simulink library "Sim_Library"  (R2015b)
settings: Solver=ode45  SolverMode=SingleTasking  StartTime=0.0  StopTime=10.0  RelTol=1e-3
undefined symbols (not defined in the file): agent, CTRL, FRAME, k, k_throttle, l, ROTOR
libraries: Sim_Library x17, vrlib x2, aerolibutil x1
(part 1 of 2)
settings Model: Creator=sgjdouth  LastModifiedBy=uos
settings DataIOCC: SaveFormat=Array
settings OptimizationCC: BlockReduction=off  BooleanDataType=off
settings DebuggingCC: SaveWithParameterizedLinksMsg=none  UnderspecifiedInitializationDetection=Classic  MergeDetectMultiDrivingBlocksExec=none  SignalResolutionControl=TryResolveAllWithWarning  StrictBusMsg=Warning
settings HardwareCC: ProdBitPerPointer=32  ProdLargestAtomicFloat=None  ProdIntDivRoundTo=Undefined  ProdEndianess=Unspecified  ProdWordSize=32  ProdHWDeviceType=32-bit Generic  TargetUnknown=on
settings GRTTargetCC: GeneratePreprocessorConditionals=Disable all
settings ConfigComp: CovModelRefEnable=Off  CovSFcnEnable=off

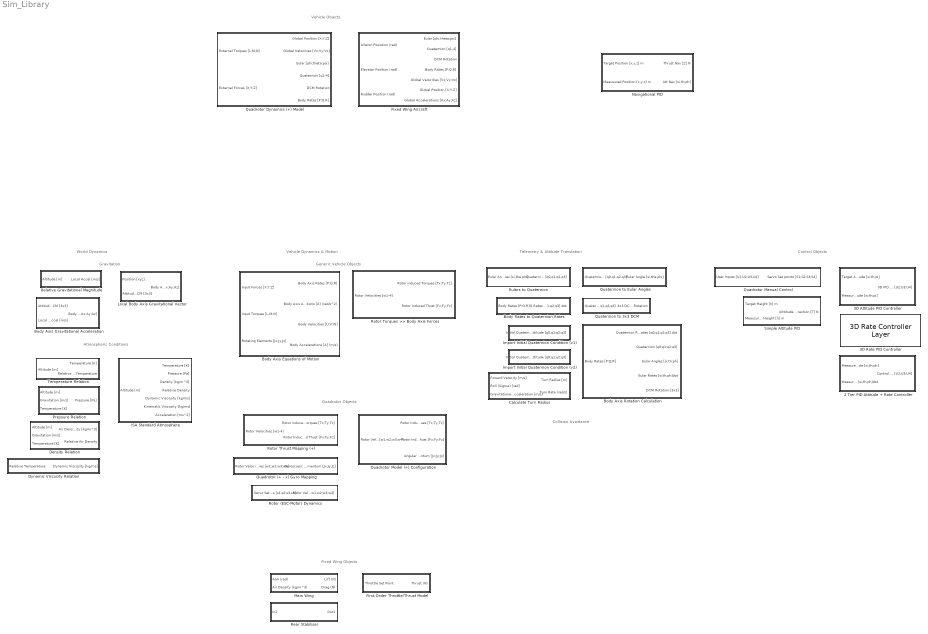
== system Sim_Library ==
  note: Gravitation
  note: Telemetry & Attitude Translation
  note: Vehicle Dynamics & Motion
  note: Control Objects
  note: World Dynamics
  note: Atmospheric Conditions
  note: Generic Vehicle Objects
  note: Quadrotor Objects
  note: Fixed Wing Objects
  note: Vehicle Objects
  note: Collision Avoidance
  2 Tier PID Attitude + Rate Controller : Subsystem
      mask Display:
      | port_label ('input',1,'IMU Attitude [\phi;\theta;\psi]','TexMode','on')
      | port_label ('input',2,'IMU Rates [\phi;\theta;\psi]dot','TexMode','on')
      | port_label ('output',1,'Control Correction [U_{2-4}]','TexMode','on')
  3D Attitude PID Controller : Subsystem
      mask Display:
      | port_label ('input',1,'Target Attitude [\phi;\theta;\psi]','TexMode','on')
      | port_label ('input',2,'Measured Attitude [\phi;\theta;\psi]','TexMode','on')
      | port_label ('output',1,'Attitude Correction [U_{2-4}]','TexMode','on')
  3D Rate PID Controller : Sim_Library/2 Tier PID Attitude + Rate Controller/3D Rate Controller Layer  SystemSampleTime=-1
  Body Axis Equations of Motion : Subsystem
      mask Display:
      | image('Sim_masks/3D_block_model.jpg')
      | port_label ('input', 1,'Net Forces [F_{x};F_{y};F_{z}]','TexMode','on')
      | port_label ('input', 2,'Net Torques [{\tau}_{L};{\tau}_{M};{\tau}_{N}]','TexMode','on')
      | port_label ('input', 3,'Rotating Elements [J_{x};J_{y};J_{z}]','TexMode','on')
      | port_label ('output',1,'Axis Rates [P;Q:R]','TexMode','on')
      | port_label ('output',2,'Angular Acceleration [omegaA]','TexMode','on')
      | port_label ('output',3,'Body Velocities [V_{x};V_{y};V_{z}]','TexMode','on')
      | port_label ('output',4,'Body Accelerations [A]','TexMode','on')
  Body Axis Gravitational Acceleration : Subsystem
      mask Display:
      | port_label ('input', 1,'Attitude DCM [3x3]','TexMode','on')
      | port_label ('input', 2,'Local Gravity [m/s]','TexMode','on')
      | port_label ('output',1,'Gravitation [g_{x};g_{y};g_{z}]','TexMode','on')
  "Body Axis Rotation Calculation " : Subsystem
      mask Display:
      | image('Sim_masks/Telemetry2.jpg')
      | port_label ('input', 1,'Body Rates [P;Q;R]','TexMode','on')
      | port_label ('output',1,'Quaternion Rates [q_{1-4}]','TexMode','on')
      | port_label ('output',2,'Quaternion [q_{1-4}]','TexMode','on')
      | port_label ('output',3,'Euler Angles [\phi;\theta;\psi]','TexMode','on')
      | port_label ('output',4,'Eular Rates [\phi;\theta;\psi]dot','TexMode','on')
      | port_label ('output',5,'DCM Rotation [3x3]')
  Body Rates to Quaternion Rates : Subsystem
      mask Display:
      | port_label ('input', 1,'Body Rates [p;q;r]','TexMode','on')
      | port_label ('output',1,'Q Rates [q_{1-4}]^{T}','TexMode','on')
  Calculate Turn Radius : Subsystem
      mask Display:
      | port_label ('input', 1,'Velocity (m/s)','TexMode','on')
      | port_label ('input', 2,'Roll Angle (rad)','TexMode','on')
      | port_label ('input', 3,'Local Gravitation (m/s)','TexMode','on')
      | port_label ('output',1,'Turn Radius (m)','TexMode','on')
      | port_label ('output',2,'Turn Rate (rad/s)','TexMode','on')
  Density Relation : Subsystem
  Dynamic Viscosity Relation : Subsystem
  Eulars to Quaternion : Subsystem
      mask Display:
      | port_label ('input', 1,'Eular Angles [\sigma;\theta;\phi]','TexMode','on')
      | port_label ('output',1,'Quaternion [q_{1-4}]^{T}','TexMode','on')
  First Order Throttle/Thrust Model : Subsystem
  Fixed Wing Aircraft : Subsystem
      mask Display:
      | image('Sim_masks/F16 wireframe.jpg');
      | port_label ('output',1,'Euler Angles [\phi;\theta;\psi]','TexMode','on');
      | port_label ('output',2,'Quaternion [q_{1-4}]','TexMode','on');
      | port_label ('output',3,'DCM Rotation [3x3]','TexMode','on');
      | port_label ('output',4,'Body Axis Rates [P;Q;R]','TexMode','on');
      | port_label ('output',5,'Velocities [V_{x},V_{y},V_{z}]','TexMode','on');
      | port_label ('output',6,'Position [x;y;z]','TexMode','on');
      | port_label ('input',1,'Velocity [V_{x};V_{y};V_{z}]','TexMode','on');
      | port_label ('input',2,'AoA (rad)','TexMode','on');
  ISA Standard Atmosphere : Subsystem
      mask Display:
      | port_label('input',1,'Altitude (m)','texmode','on')
      | port_label('output',1,'Temperature (K)','texmode','on')
      | port_label('output',2,'Pressure (Pa)','texmode','on')
      | port_label('output',3,'Density (kg/m^3)','texmode','on')
      | port_label('output',4,'Relative Density','texmode','on')
      | port_label('output',5,'Dynamic Viscosity (kg/ms)','texmode','on')
      | port_label('output',6,'Kinematic Viscosity (kg/ms)','texmode','on')
      | port_label('output',7,'Acceleration (ms^2)','texmode','on')
  Import Initial Quaternion Condition (v1) : Subsystem
      mask Display: port_label ('output',1,'Initial Quaternion [q_{1-4}]^{T}','TexMode','on')
  Import Initial Quaternion Condition (v2) : Subsystem
      mask Display: port_label ('output',1,'Initial Quaternion [q_{1-4}]^{T}','TexMode','on')
  Local Body Axis Gravitational Vector : Subsystem
      mask Display:
      | port_label ('input', 1,'Position [X;Y;Z]','TexMode','on')
      | port_label ('input', 2,'Attitude DCM [3x3]','TexMode','on')
      | port_label ('output',1,'Body Gravitation [g_{x};g_{y};g_{z}]','TexMode','on')
  "Main Wing " : Subsystem
  Navigational PID : Subsystem
  Pressure Relation : Subsystem
  Quadrotor (+ - x) Gyro Mapping : Subsystem
      mask Display:
      | port_label ('input', 1,'Rotor Velocities [{\omega}_{1-4}]^{T}','TexMode','on')
      | port_label ('output',1,'Rotor Momentum [J_{x};J_{y};J_{z}]','TexMode','on')
  Quadrotor Dynamics (+) Model : Subsystem
      mask Display:
      | image('Sim_masks/QuadMask+.jpg');
      | port_label ('output',1,'Euler Angles [\phi;\theta;\psi]','TexMode','on');
      | port_label ('output',2,'Quaternion [q_{1-4}]','TexMode','on');
      | port_label ('output',3,'DCM Rotation [3x3]','TexMode','on');
      | port_label ('output',4,'Body Axis Rates [P;Q;R]','TexMode','on');
      | port_label ('output',5,'Velocities [V_{x},V_{y},V_{z}]','TexMode','on');
      | port_label ('output',6,'Position [x;y;z]','TexMode','on');
      | port_label ('input',1,'Rotor Velocities [\omega_{1-4}]','TexMode','on');
      | port_label ('input',2,'External Torques [L;M;N]','TexMode','on');
      | port_label ('input',3,'External Forces [F_{x};F_{y};F_{z}]','TexMode','on');
  "Quadrotor Manual Control " : Subsystem
      mask Display:
      | port_label ('input',1,'Control Inputs [U_{1-4}]','TexMode','on')
      | port_label ('output',1,'Servo Set Points_{0-255} [S_{1-4}]','TexMode','on')
  Quadrotor Model (+) Configuration : Subsystem
      mask Display:
      | port_label ('input', 1,'Rotor Velocities [\omega_{1-4}]','TexMode','on')
      | port_label ('output',1,'Net Torques [\tau_{x},\tau_{y},\tau_{z}]','TexMode','on')
      | port_label ('output',2,'Net Thrust [F_{x},F_{y},F_{z}]','TexMode','on')
      | port_label ('output',3,'Angular Momentum [J_{x},J_{y},J_{z}]','TexMode','on')
  "Quaternion to 3x3 DCM " : Subsystem
      mask Display:
      | port_label ('input', 1,'Quaternion [q_{1-4}]^{T}','TexMode','on')
      | port_label ('output',1,'DCM [3x3]','TexMode','on')
  Quaternion to Eular Angles : Subsystem
      mask Display:
      | port_label ('input',1,'Quaternion [q_{1-4}]^{T}','TexMode','on')
      | port_label ('output',1,'Eular Angles [\sigma;\theta;\phi]','TexMode','on')
  Rear Stabiliser : Subsystem
  Relative Gravitational Magnitude : Subsystem
  Rotor (ESC-Motor) Dynamics : Subsystem
      mask Display:
      | port_label ('input', 1,'Servo CMD [S_{1-4}]','TexMode','on')
      | port_label ('output',1,'Rotational Rates [\omega_{1-4}]','TexMode','on')
  Rotor Thrust Mapping (+) : Subsystem
      mask Display:
      | port_label ('input', 1,'Rotor Velocities [\omega_{1-4}]','TexMode','on')
      | port_label ('output',1,'Rotor Induced Torques [\tau_{x},\tau_{y},\tau_{z}]','TexMode','on')
      | port_label ('output',2,'Rotor Induced Thrust [F_{x},F_{y},F_{z}]','TexMode','on')
  Rotor Torques >> Body Axis Forces : Subsystem
      mask Display:
      | image('Sim_masks/Body Arm Coordinates.jpg')
      | port_label ('input', 1,'Rotor Velocities [\omega_{1-N}]','TexMode','on')
      | port_label ('output',1,'Rotor Induced Torques [\tau_{x},\tau_{y},\tau_{z}]','TexMode','on')
      | port_label ('output',2,'Rotor Induced Thrust [F_{x},F_{y},F_{z}]','TexMode','on')
  Simple Altitude PID : Subsystem
      mask Display:
      | port_label ('input',1,'Target Altitude [m]','TexMode','on')
      | port_label ('input',2,'Measured Altitude [m]','TexMode','on')
      | port_label ('output',1,'Throttle Correction [U_{1}]','TexMode','on')
  Temperature Relation : Subsystem

== system Sim_Library/2 Tier PID Attitude + Rate Controller ==
  Measured Attitude [si;th;ph] : Inport
  Measured Rates [si;th;ph]dot : Inport  Port=2
  3D PID Controller (Attitude) : Sim_Library/3D PID Controller (Attitude)
  3D Rate Controller Layer : Subsystem
      mask Display:
      | port_label ('input',1,'Measured Rates [\phi;\theta;\psi]dot','TexMode','on')
      | port_label ('input',2,'Target Rates [\phi;\theta;\psi]dot','TexMode','on')
      | port_label ('output',1,'Attitude Correction [U_{2-4}]','TexMode','on')
  Hold Level Horizon : Constant  Value=[0;0;0]
  Control Outputs [U2;U3;U4] : Outport
  wires:
  3D Rate Controller Layer/1(PID Outputs [Ksi;Kth;Kpi]) -> Control Outputs [U2;U3;U4]/1
  Measured Rates [si;th;ph]dot/1 -> 3D Rate Controller Layer/1(Measured Rates [si;th;pi] dot)
  3D PID Controller (Attitude)/1 -> 3D Rate Controller Layer/2(Target Rates [si;th;pi] dot)
  Hold Level Horizon/1 -> 3D PID Controller (Attitude)/1
  Measured Attitude [si;th;ph]/1 -> 3D PID Controller (Attitude)/2

== system Sim_Library/3D Attitude PID Controller ==
  note: 3D PID Attitude Control Calculator
  Target Attitude [si;th;pi] : Inport
  Measured Attitude [si;th;pi] : Inport  Port=2
  Attitude Integrator : Integrator  InitialCondition=[0;0;0]
  Constant : Constant  Value=CTRL.kp  VectorParams1D=off
  Constant1 : Constant  Value=CTRL.kd  VectorParams1D=off
  Constant2 : Constant  Value=CTRL.ki  VectorParams1D=off
  D Gains [si,th,pi] : Product
  Derivative : Derivative
  Display : Display
  Display1 : Display
  I Gains [si,th,pi] : Product
  P Gains [si,th,pi] : Product
  Subtract : Sum  Inputs=-+
  Sum2 : Sum  Inputs=+++
  3D PID Outputs [U2;U3;U4] : Outport
  wires:
  Target Attitude [si;th;pi]/1 -> Subtract/2
  Measured Attitude [si;th;pi]/1 -> Display1/1, Subtract/1
  Sum2/1 -> 3D PID Outputs [U2;U3;U4]/1, Display/1
  Derivative/1 -> Sum2/3
  Subtract/1 -> D Gains [si,th,pi]/2, P Gains [si,th,pi]/2, I Gains [si,th,pi]/2
  Constant1/1 -> D Gains [si,th,pi]/1
  Constant/1 -> P Gains [si,th,pi]/1
  Constant2/1 -> I Gains [si,th,pi]/1
  D Gains [si,th,pi]/1 -> Derivative/1
  P Gains [si,th,pi]/1 -> Sum2/1
  Attitude Integrator/1 -> Sum2/2
  I Gains [si,th,pi]/1 -> Attitude Integrator/1

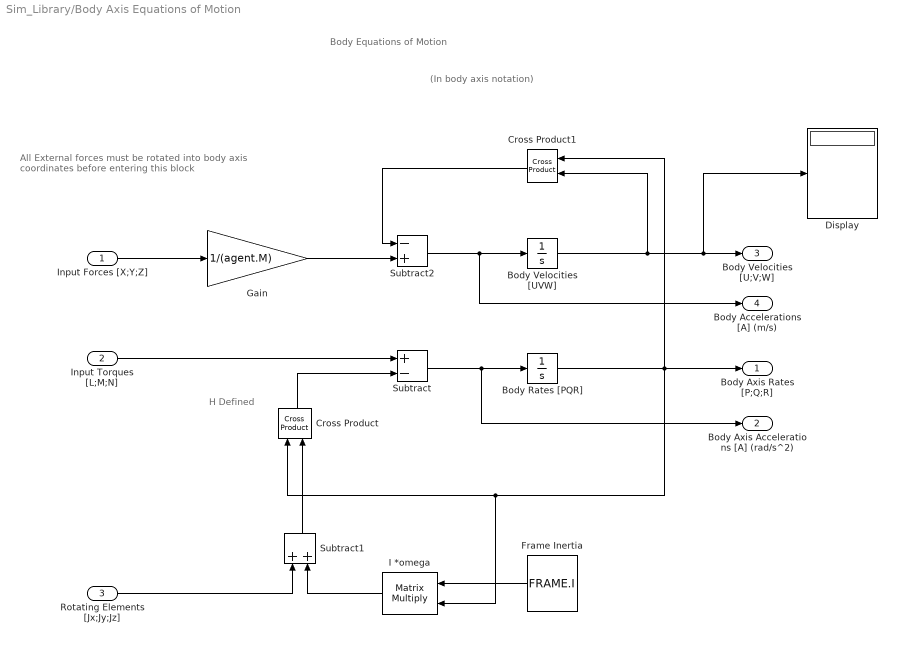
== system Sim_Library/Body Axis Equations of Motion ==
  note: All External forces must be rotated into
      | body axis coordinates before entering this block
  note: (In body axis notation)
  note: Body Equations of Motion
  note: H Defined
  Input Forces [X;Y;Z] : Inport
  Input Torques [L;M;N] : Inport  Port=2
  Rotating Elements [Jx;Jy;Jz] : Inport  Port=3
  Body Rates [PQR] : Integrator  InitialCondition=[0;0;0]
  Body Velocities [UVW] : Integrator  InitialCondition=[0;0;0]
  Cross Product : vrlib/Utilities/Cross Product
  Cross Product1 : vrlib/Utilities/Cross Product
  Display : Display
  Frame Inertia : Constant  Value=FRAME.I
  Gain : Gain  Gain=1/(agent.M)
  I *omega : Product  Multiplication=Matrix(*)
  Subtract : Sum  Inputs=+-
  Subtract1 : Sum
  Subtract2 : Sum  Inputs=-+
  Body Axis Rates [P;Q;R] : Outport
  Body Axis Accelerations [A] (rad/s^2) : Outport  Port=2
  Body Velocities [U;V;W] : Outport  Port=3
  Body Accelerations [A] (m/s) : Outport  Port=4
  wires:
  Gain/1 -> Subtract2/2
  Subtract2/1 -> Body Accelerations [A] (m/s)/1, Body Velocities [UVW]/1
  Cross Product1/1 -> Subtract2/1
  Body Velocities [UVW]/1 -> Display/1, Body Velocities [U;V;W]/1, Cross Product1/2
  Body Rates [PQR]/1 -> I *omega/2, Cross Product/1, Body Axis Rates [P;Q;R]/1, Cross Product1/1
  Frame Inertia/1 -> I *omega/1
  Subtract/1 -> Body Axis Accelerations [A] (rad/s^2)/1, Body Rates [PQR]/1
  Cross Product/1 -> Subtract/2
  I *omega/1 -> Subtract1/2
  Subtract1/1 -> Cross Product/2
  Input Forces [X;Y;Z]/1 -> Gain/1
  Input Torques [L;M;N]/1 -> Subtract/1
  Rotating Elements [Jx;Jy;Jz]/1 -> Subtract1/1

== system Sim_Library/Body Axis Gravitational Acceleration ==
  note: Gravitational Model
  note: Newtons equation of gravity, extended to provide a local gravitational vector
  note: Assumptions; Gravitational linearity, reference is Earth and down is positive.
  Attitude DCM [3x3] : Inport
  Local Gravitational Accel [m/s] : Inport  Port=2
  Gain : Gain  Gain=[0;0;1]
  Product1 : Product  Multiplication=Matrix(*)
  Body Accel [Ax;Ay;Az] : Outport
  wires:
  Gain/1 -> Product1/2
  Product1/1 -> Body Accel [Ax;Ay;Az]/1
  Attitude DCM [3x3]/1 -> Product1/1
  Local Gravitational Accel [m/s]/1 -> Gain/1

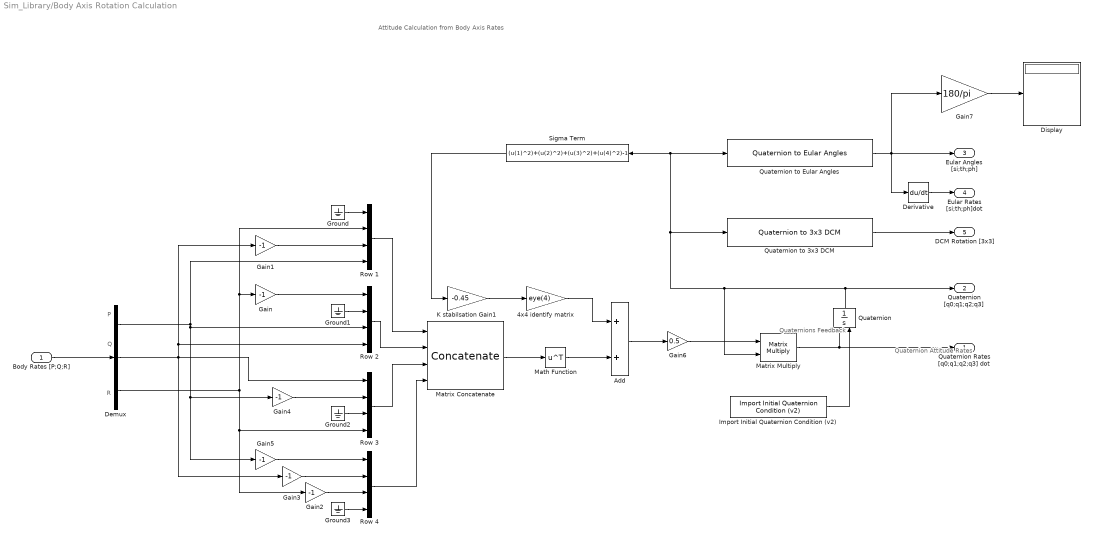
== system Sim_Library/Body Axis Rotation Calculation  ==
  note: R
  note: Q
  note: P
  note: Quaternions Feedback
  note: Attitude Calculation from Body Axis Rates
  note: Quaternion Attitude Rates
  Body Rates [P;Q;R] : Inport
  4x4 identify matrix : Gain  Gain=eye(4)
  Add : Sum
  Demux : Demux  Outputs=3
  Derivative : Derivative
  Display : Display
  Gain{,1..5} (6 alike) : Gain  Gain=-1
  Gain6 : Gain  Gain=0.5
  Gain7 : Gain  Gain=180/pi
  Ground{,1..3} (4 alike) : Ground
  Import Initial Quaternion Condition (v2) : Sim_Library/Import Initial Quaternion Condition (v2)  SystemSampleTime=-1
  K stabilsation Gain1 : Gain  Gain=-0.45
  Math Function : Math  Operator=transpose  SaturateOnIntegerOverflow=on
  Matrix Concatenate : Concatenate  NumInputs=4  Mode=Multidimensional array  ConcatenateDimension=2
  Matrix Multiply : Product  Multiplication=Matrix(*)
  Quaternion : Integrator  InitialConditionSource=external  InitialCondition=[0;0;0;1]  ZeroCross=off
  "Quaternion to 3x3 DCM " : Sim_Library/Quaternion to 3x3 DCM   SystemSampleTime=-1
  Quaternion to Eular Angles : Sim_Library/Quaternion to Eular Angles  SystemSampleTime=-1
  Row {1..4} (4 alike) : Concatenate  NumInputs=4
  Sigma Term : Fcn  Expr=(u(1)^2)+(u(2)^2)+(u(3)^2)+(u(4)^2)-1
  Quaternion Rates [q0;q1;q2;q3] dot : Outport
  Quaternion [q0;q1;q2;q3] : Outport  Port=2
  Eular Angles [si;th;ph] : Outport  Port=3
  Eular Rates [si;th;ph]dot : Outport  Port=4
  DCM Rotation [3x3] : Outport  Port=5
  wires:
  Math Function/1 -> Add/2
  Body Rates [P;Q;R]/1 -> Demux/1
  Gain7/1 -> Display/1
  K stabilsation Gain1/1 -> 4x4 identify matrix/1
  Add/1 -> Gain6/1
  4x4 identify matrix/1 -> Add/1
  Matrix Concatenate/1 -> Math Function/1
  Ground1/1 -> Row 2/2
  Ground2/1 -> Row 3/3
  Ground3/1 -> Row 4/4
  Ground/1 -> Row 1/1
  Gain5/1 -> Row 4/1
  Gain4/1 -> Row 3/2
  Demux/1 -> Row 2/3, Gain4/1, Gain5/1, Row 1/4
  Gain3/1 -> Row 4/2
  Gain1/1 -> Row 1/3
  Demux/2 -> Gain3/1, Row 3/1, Row 2/4, Gain1/1
  Gain2/1 -> Row 4/3
  Gain/1 -> Row 2/1
  Demux/3 -> Row 3/4, Gain2/1, Row 1/2, Gain/1
  Row 1/1 -> Matrix Concatenate/1
  Row 2/1 -> Matrix Concatenate/2
  Row 3/1 -> Matrix Concatenate/3
  Row 4/1 -> Matrix Concatenate/4
  Matrix Multiply/1 -> Quaternion Rates [q0;q1;q2;q3] dot/1, Quaternion/1
  Sigma Term/1 -> K stabilsation Gain1/1
  Gain6/1 -> Matrix Multiply/1
  Quaternion/1 -> Quaternion [q0;q1;q2;q3]/1, Quaternion to Eular Angles/1, Sigma Term/1, "Quaternion to 3x3 DCM "/1, Matrix Multiply/2
  "Quaternion to 3x3 DCM "/1 -> DCM Rotation [3x3]/1
  Quaternion to Eular Angles/1 -> Gain7/1, Derivative/1, Eular Angles [si;th;ph]/1
  Derivative/1 -> Eular Rates [si;th;ph]dot/1
  Import Initial Quaternion Condition (v2)/1 -> Quaternion/2

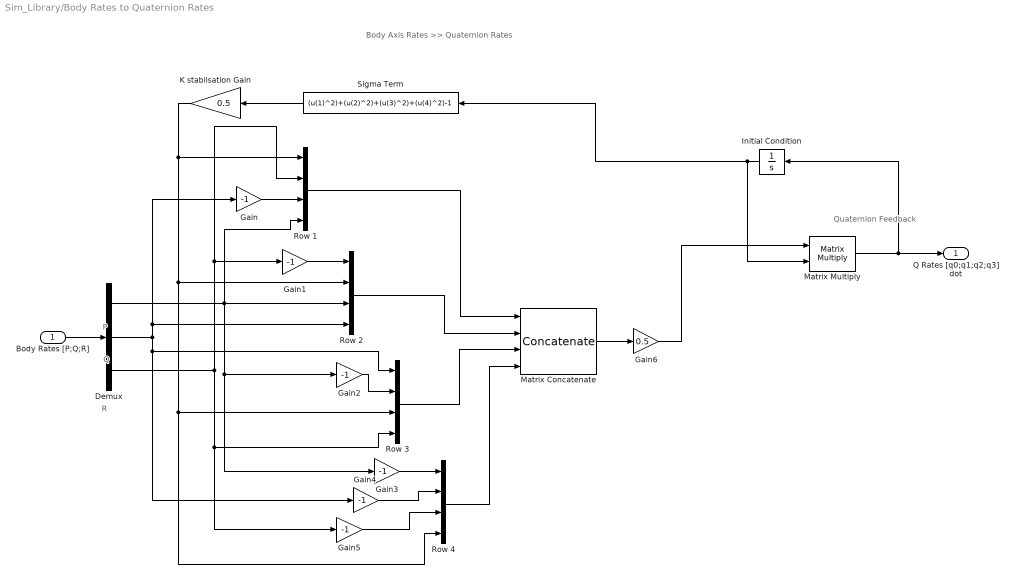
== system Sim_Library/Body Rates to Quaternion Rates ==
  note: Quaternion Feedback
  note: P
  note: Q
  note: R
  note: Body Axis Rates >> Quaternion Rates
  Body Rates [P;Q;R] : Inport
  Demux : Demux  Outputs=3
  Gain{,1..5} (6 alike) : Gain  Gain=-1
  Gain6 : Gain  Gain=0.5
  "Initial Condition " : Integrator  InitialCondition=[0;0;0]
  K stabilsation Gain : Gain  Gain=0.5
  Matrix Concatenate : Concatenate  NumInputs=4  Mode=Multidimensional array  ConcatenateDimension=2
  Matrix Multiply : Product  Multiplication=Matrix(*)
  Row {1..4} (4 alike) : Concatenate  NumInputs=4
  Sigma Term : Fcn  Expr=(u(1)^2)+(u(2)^2)+(u(3)^2)+(u(4)^2)-1
  Q Rates [q0;q1;q2;q3] dot : Outport
  wires:
  "Initial Condition "/1 -> Sigma Term/1, Matrix Multiply/2
  Gain6/1 -> Matrix Multiply/1
  K stabilsation Gain/1 -> Row 1/1, Row 2/2, Row 3/3, Row 4/4
  Sigma Term/1 -> K stabilsation Gain/1
  Matrix Multiply/1 -> Q Rates [q0;q1;q2;q3] dot/1, "Initial Condition "/1
  Matrix Concatenate/1 -> Gain6/1
  Row 4/1 -> Matrix Concatenate/4
  Row 3/1 -> Matrix Concatenate/3
  Row 2/1 -> Matrix Concatenate/2
  Row 1/1 -> Matrix Concatenate/1
  Gain5/1 -> Row 4/3
  Gain4/1 -> Row 4/2
  Gain3/1 -> Row 4/1
  Gain2/1 -> Row 3/2
  Gain1/1 -> Row 2/1
  Demux/1 -> Row 1/4, Row 2/3, Gain2/1, Gain3/1
  Demux/2 -> Gain/1, Row 2/4, Gain4/1, Row 3/1
  Gain/1 -> Row 1/3
  Demux/3 -> Gain1/1, Row 1/2, Row 3/4, Gain5/1
  Body Rates [P;Q;R]/1 -> Demux/1

== system Sim_Library/Calculate Turn Radius ==
  note: Turn Radius, R = V^2/(g*tan(sig))
  note: Calculate Turn Performance Parameters
  note: Yaw rate, Phi = (g*tan(sig))/V
  Foward Velocity [m/s] : Inport
  Roll (Sigma) [rad] : Inport  Port=2
  Gravitational Acceleration [m/s] : Inport  Port=3
  (g*tan(sig))/V : Product  Inputs=*/
  V^2 : Math  Operator=square  SaturateOnIntegerOverflow=on
  V^2/(g*tan(sig) : Product  Inputs=*/
  g*tan(sig) : Product
  tan(sig) : Trigonometry  Operator=tan
  Turn Radius [m] : Outport
  Turn Rate (rad/s) : Outport  Port=2
  wires:
  Foward Velocity [m/s]/1 -> (g*tan(sig))/V/2, V^2/1
  V^2/1 -> V^2/(g*tan(sig)/1
  Roll (Sigma) [rad]/1 -> tan(sig)/1
  tan(sig)/1 -> g*tan(sig)/1
  Gravitational Acceleration [m/s]/1 -> g*tan(sig)/2
  g*tan(sig)/1 -> V^2/(g*tan(sig)/2, (g*tan(sig))/V/1
  V^2/(g*tan(sig)/1 -> Turn Radius [m]/1
  (g*tan(sig))/V/1 -> Turn Rate (rad/s)/1

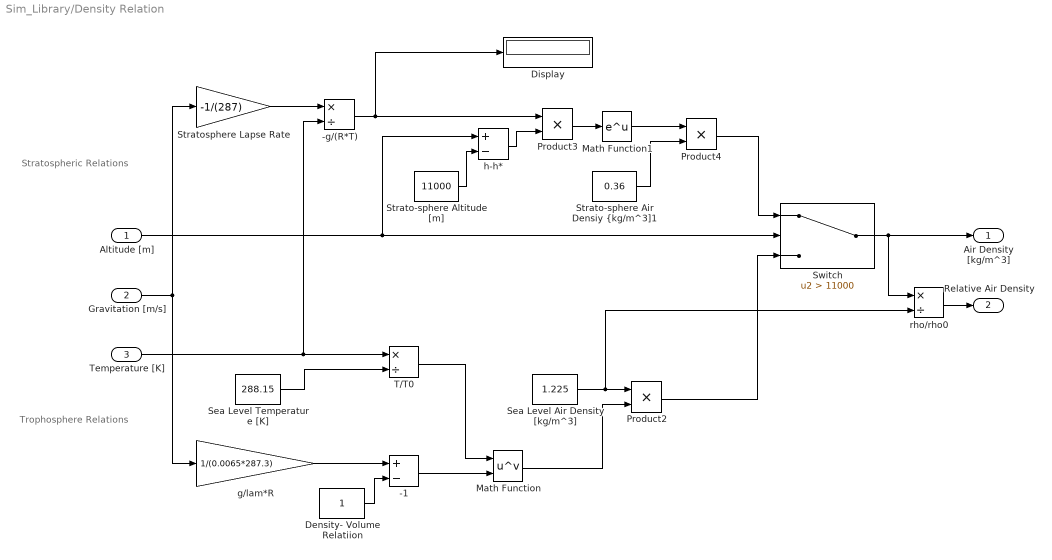
== system Sim_Library/Density Relation ==
  note: Trophosphere Relations
  note: Stratospheric Relations
  Altitude [m] : Inport
  Gravitation [m/s] : Inport  Port=2
  Temperature [K] : Inport  Port=3
  -1 : Sum  Inputs=+-
  -g/(R*T) : Product  Inputs=*/
  Density- Volume Relatiion : Constant
  Display : Display
  Math Function : Math  Operator=pow  SaturateOnIntegerOverflow=on
  Math Function1 : Math  SaturateOnIntegerOverflow=on
  Product2 : Product
  Product3 : Product
  Product4 : Product
  Sea Level Temperature [K] : Constant  Value=288.15
  Sea Level Air Density [kg/m^3] : Constant  Value=1.225
  Strato-sphere Altitude [m] : Constant  Value=11000
  "Strato-sphere Air Densiy {kg/m^3]1" : Constant  Value=0.36
  Stratosphere Lapse Rate : Gain  Gain=-1/(287)
  Switch : Switch  Criteria=u2 > Threshold  Threshold=11000
  T/T0 : Product  Inputs=*/
  g/lam*R : Gain  Gain=1/(0.0065*287.3)
  h-h* : Sum  Inputs=+-
  rho/rho0 : Product  Inputs=*/
  Air Density [kg/m^3] : Outport
  Relative Air Density : Outport  Port=2
  wires:
  -1/1 -> Math Function/2
  Switch/1 -> Air Density [kg/m^3]/1, rho/rho0/1
  Altitude [m]/1 -> h-h*/1, Switch/2
  Gravitation [m/s]/1 -> g/lam*R/1, Stratosphere Lapse Rate/1
  Temperature [K]/1 -> -g/(R*T)/2, T/T0/1
  Sea Level Temperature [K]/1 -> T/T0/2
  T/T0/1 -> Math Function/1
  Sea Level Air Density [kg/m^3]/1 -> rho/rho0/2, Product2/1
  Math Function/1 -> Product2/2
  Product2/1 -> Switch/3
  Strato-sphere Altitude [m]/1 -> h-h*/2
  h-h*/1 -> Product3/2
  Product3/1 -> Math Function1/1
  Math Function1/1 -> Product4/1
  "Strato-sphere Air Densiy {kg/m^3]1"/1 -> Product4/2
  Product4/1 -> Switch/1
  g/lam*R/1 -> -1/1
  Density- Volume Relatiion/1 -> -1/2
  Stratosphere Lapse Rate/1 -> -g/(R*T)/1
  -g/(R*T)/1 -> Product3/1, Display/1
  rho/rho0/1 -> Relative Air Density/1

== system Sim_Library/Dynamic Viscosity Relation ==
  Relative Temperature : Inport
  Display1 : Display
  Dynamic Viscosity Lapse Rate : Constant  Value=3/4
  "Sea Level Dynamic Viscosity " : Constant  Value=1.78E-05
  exp2 : Math  Operator=pow  SaturateOnIntegerOverflow=on
  mu0 *(T/T0) : Product
  Dynamic Viscosity [kg/ms] : Outport
  wires:
  Relative Temperature/1 -> mu0 *(T/T0)/1
  mu0 *(T/T0)/1 -> exp2/1
  Dynamic Viscosity Lapse Rate/1 -> exp2/2
  exp2/1 -> Dynamic Viscosity [kg/ms]/1, Display1/1
  "Sea Level Dynamic Viscosity "/1 -> mu0 *(T/T0)/2

== system Sim_Library/Eulars to Quaternion ==
  note: Eular Angles >> Quaternions
  Eular Angles [si,the,phi] : Inport
  Definition of q0 : Fcn  Expr=cos(u(1)/2)*cos(u(2)/2)*cos(u(3)/2)+sin(u(1)/2)*sin(u(2)/2)*sin(u(3)/2)
  Definition of q1 : Fcn  Expr=sin(u(1)/2)*cos(u(2)/2)*cos(u(3)/2)-cos(u(1)/2)*sin(u(2)/2)*sin(u(3)/2)
  Definition of q2 : Fcn  Expr=cos(u(1)/2)*sin(u(2)/2)*cos(u(3)/2)+sin(u(1)/2)*cos(u(2)/2)*sin(u(3)/2)
  Definition of q3 : Fcn  Expr=cos(u(1)/2)*cos(u(2)/2)*sin(u(3)/2)-sin(u(1)/2)*sin(u(2)/2)*cos(u(3)/2)
  Vector Concatenate : Concatenate  NumInputs=4  Mode=Multidimensional array
  Quaternion [q0,q1,q2,q3] : Outport
  wires:
  Definition of q0/1 -> Vector Concatenate/1
  Definition of q1/1 -> Vector Concatenate/2
  Definition of q2/1 -> Vector Concatenate/3
  Definition of q3/1 -> Vector Concatenate/4
  Vector Concatenate/1 -> Quaternion [q0,q1,q2,q3]/1
  Eular Angles [si,the,phi]/1 -> Definition of q0/1, Definition of q1/1, Definition of q3/1, Definition of q2/1

== system Sim_Library/First Order Throttle//Thrust Model ==
  note: Details given on page 51, Cook 2007
  note: Simple First Order Engine Approximation
  "Throttle Set Point " : Inport
  First order lag transfer function : TransferFcn  Denominator=[2.5 1]
  Gain : Gain  Gain=k_throttle
  Thrust (N) : Outport
  wires:
  "Throttle Set Point "/1 -> Gain/1
  Gain/1 -> First order lag transfer function/1
  First order lag transfer function/1 -> Thrust (N)/1

== system Sim_Library/Fixed Wing Aircraft ==
  note: Calculation of the aircraft specific forces
  note: Translate body axes vectors into earth axes
  note: Fixed Wing Dynamic Model
  Aileron Posistion (rad) : Inport
  Elevator Position (rad) : Inport  Port=2
  Rudder Position (rad) : Inport  Port=3
  Body Axis Equations of Motion : Sim_Library/Body Axis Equations of Motion  SystemSampleTime=-1
  "Body Axis Rotation Calculation " : Sim_Library/Body Axis Rotation Calculation   SystemSampleTime=-1
  Derivative : Derivative
  Integrator : Integrator  InitialCondition=[0;0;0]
  Product1 : Product  Multiplication=Matrix(*)
  Terminator : Terminator
  Terminator1 : Terminator
  Eular [phi;theta;psi] : Outport
  Quaternion [q1-4] : Outport  Port=2
  DCM Rotation : Outport  Port=3
  Body Rates [P;Q;R] : Outport  Port=4
  Global Velocities [Vx;Vy;Vz] : Outport  Port=5
  Global Position [X;Y;Z] : Outport  Port=6
  Global Accelerations [Ax;Ay;Az] : Outport  Port=7
  wires:
  Body Axis Equations of Motion/1 -> Body Rates [P;Q;R]/1, "Body Axis Rotation Calculation "/1
  "Body Axis Rotation Calculation "/3 -> Eular [phi;theta;psi]/1
  "Body Axis Rotation Calculation "/2 -> Quaternion [q1-4]/1
  Integrator/1 -> Global Position [X;Y;Z]/1
  "Body Axis Rotation Calculation "/1 -> Terminator/1
  "Body Axis Rotation Calculation "/4 -> Terminator1/1
  Product1/1 -> Integrator/1, Derivative/1, Global Velocities [Vx;Vy;Vz]/1
  "Body Axis Rotation Calculation "/5 -> Product1/1, DCM Rotation/1
  Body Axis Equations of Motion/3 -> Product1/2
  Derivative/1 -> Global Accelerations [Ax;Ay;Az]/1

== system Sim_Library/ISA Standard Atmosphere ==
  note: This module is designed to emulate the International Standard Atmosphere (ISA) on Earth
  note: ISA Atmospheric Model
  Altitude [m] : Inport
  Density Relation : Sim_Library/Density Relation
  Dynamic Viscosity Relation : Sim_Library/Dynamic Viscosity Relation
  Pressure Relation : Sim_Library/Pressure Relation
  Relative Gravitational Magnitude : Sim_Library/Relative Gravitational Magnitude
  Temperature Relation : Sim_Library/Temperature Relation
  mu/rho : Product  Inputs=*/
  Temperature [K] : Outport
  Pressure [Pa] : Outport  Port=2
  Density [kg/m^3] : Outport  Port=3
  Relative Density : Outport  Port=4
  Dynamic Viscosity [kg/ms] : Outport  Port=5
  Kinematic Viscosity [kg/ms] : Outport  Port=6
  Acceleration [ms^2] : Outport  Port=7
  wires:
  Relative Gravitational Magnitude/1 -> Acceleration [ms^2]/1, Density Relation/2, Pressure Relation/2
  Altitude [m]/1 -> Density Relation/1, Pressure Relation/1, Temperature Relation/1, Relative Gravitational Magnitude/1
  Density Relation/2 -> Relative Density/1
  Density Relation/1 -> mu/rho/2, Density [kg/m^3]/1
  Temperature Relation/2 -> Dynamic Viscosity Relation/1
  Dynamic Viscosity Relation/1 -> mu/rho/1, Dynamic Viscosity [kg/ms]/1
  mu/rho/1 -> Kinematic Viscosity [kg/ms]/1
  Pressure Relation/1 -> Pressure [Pa]/1
  Temperature Relation/1 -> Density Relation/3, Pressure Relation/3, Temperature [K]/1

== system Sim_Library/Import Initial Quaternion Condition (v1) ==
  note: Input angle is declared as :
      | agent.intial_attitude
  note: Initial input angle to be defined in
      | the workspace for a generic agent.
      |
      | Workspace initial angle is given as a
      | Eular array, however must be converted
      | to a quaternion before fed into the system.
  note: Initial Eular Condition >> Quaternion Input Conditions
  Mux : Mux
  q0 : Constant  Value=(cos(agent.initial_attitude(1)/2)*cos(agent.initial_attitude(2)/2)*cos(agent.initial_attitude(3)/2)+sin(agent.initial_attitude(1)/2)*sin(agent.initial_attitude(2)/2)*sin(agent.initial_attitude(3)/2))
  q1 : Constant  Value=(sin(agent.initial_attitude(1)/2)*cos(agent.initial_attitude(2)/2)*cos(agent.initial_attitude(3)/2)-cos(agent.initial_attitude(1)/2)*sin(agent.initial_attitude(2)/2)*sin(agent.initial_attitude(3)/2))
  q2 : Constant  Value=(cos(agent.initial_attitude(1)/2)*sin(agent.initial_attitude(2)/2)*cos(agent.initial_attitude(3)/2)+sin(agent.initial_attitude(1)/2)*cos(agent.initial_attitude(2)/2)*sin(agent.initial_attitude(3)/2))
  q3 : Constant  Value=(cos(agent.initial_attitude(1)/2)*cos(agent.initial_attitude(2)/2)*sin(agent.initial_attitude(3)/2)-sin(agent.initial_attitude(1)/2)*sin(agent.initial_attitude(2)/2)*cos(agent.initial_attitude(3)/2))
  Initial Quaternion Attitude [q0;q1;q2;q3] : Outport
  wires:
  q0/1 -> Mux/4
  q3/1 -> Mux/3
  q2/1 -> Mux/2
  q1/1 -> Mux/1
  Mux/1 -> Initial Quaternion Attitude [q0;q1;q2;q3]/1

== system Sim_Library/Import Initial Quaternion Condition (v2) ==
  note: Input variable defined in the workspace as:
      | agent.initial_attitude
  note: Initial Eular Condition >> Quaternion Input Conditions
  note: Initial input angle to be defined in
      | the workspace for a generic agent.
      | Workspace initial angle is given as a
      | Eular array, however must be converted
      | to a quaternion before fed into the system.
  Constant from workspace : Constant  Value=agent.initial_attitude
  Fcn : Fcn  Expr=(sin(u(1)/2)*cos(u(2)/2)*cos(u(3)/2)-cos(u(1)/2)*sin(u(2)/2)*sin(u(3)/2))
  Fcn1 : Fcn  Expr=(cos(u(1)/2)*sin(u(2)/2)*cos(u(3)/2)+sin(u(1)/2)*cos(u(2)/2)*sin(u(3)/2))
  Fcn2 : Fcn  Expr=(cos(u(1)/2)*cos(u(2)/2)*sin(u(3)/2)-sin(u(1)/2)*sin(u(2)/2)*cos(u(3)/2))
  Fcn3 : Fcn  Expr=(cos(u(1)/2)*cos(u(2)/2)*cos(u(3)/2)+sin(u(1)/2)*sin(u(2)/2)*sin(u(3)/2))
  Mux1 : Mux
  Initial Quaternion Attitude [q0;q1;q2;q3] : Outport
  wires:
  Constant from workspace/1 -> Fcn/1, Fcn1/1, Fcn2/1, Fcn3/1
  Mux1/1 -> Initial Quaternion Attitude [q0;q1;q2;q3]/1
  Fcn/1 -> Mux1/1
  Fcn1/1 -> Mux1/2
  Fcn2/1 -> Mux1/3
  Fcn3/1 -> Mux1/4

== system Sim_Library/Local Body Axis Gravitational Vector ==
  note: Gravitational Model (vector)
  note: Newtons equation of gravity, extended to provide a local gravitational vector
  note: Assumptions; Gravitational linearity, reference is Earth and down is positive.
  note: Acceleration as a
      | global constant
  Position [xyz] : Inport
  Attitude DCM [3x3] : Inport  Port=2
  Demux : Demux  Outputs=3
  Divide : Product  Inputs=*/
  Gain : Gain  Gain=[0;0;1]
  Gravitational Constant [Nm^2/kg^2] : Constant  Value=6.673*10^-11  VectorParams1D=off
  Mass Of The Earth [kg] : Constant  Value=5.972*10^24  VectorParams1D=off
  Math Function : Math  Operator=square  SaturateOnIntegerOverflow=on
  Product : Product
  Product1 : Product  Multiplication=Matrix(*)
  Radius of The Earth [m] : Constant  Value=6371*10^3  VectorParams1D=off
  Sum : Sum  Inputs=|++
  Terminator : Terminator
  Terminator1 : Terminator
  Body Accel [Ax;Ay;Az] : Outport
  wires:
  Math Function/1 -> Divide/2
  Product/1 -> Divide/1
  Sum/1 -> Math Function/1
  Radius of The Earth [m]/1 -> Sum/2
  Mass Of The Earth [kg]/1 -> Product/2
  Gravitational Constant [Nm^2/kg^2]/1 -> Product/1
  Gain/1 -> Product1/2
  Attitude DCM [3x3]/1 -> Product1/1
  Divide/1 -> Gain/1
  Product1/1 -> Body Accel [Ax;Ay;Az]/1
  Position [xyz]/1 -> Demux/1
  Demux/3 -> Sum/1
  Demux/1 -> Terminator/1
  Demux/2 -> Terminator1/1

== system Sim_Library/Main Wing  ==
  AoA (rad) : Inport
  Air Density (kg/m^3) : Inport  Port=2
  Get chord length : FromWorkspace  VariableName=agent.main_wing_chord  SampleTime=0
  Get main wing lift coefficient : FromWorkspace  VariableName=agent.main_wing_cl  SampleTime=0
  Lift (N) : Outport
  Drag (N) : Outport  Port=2

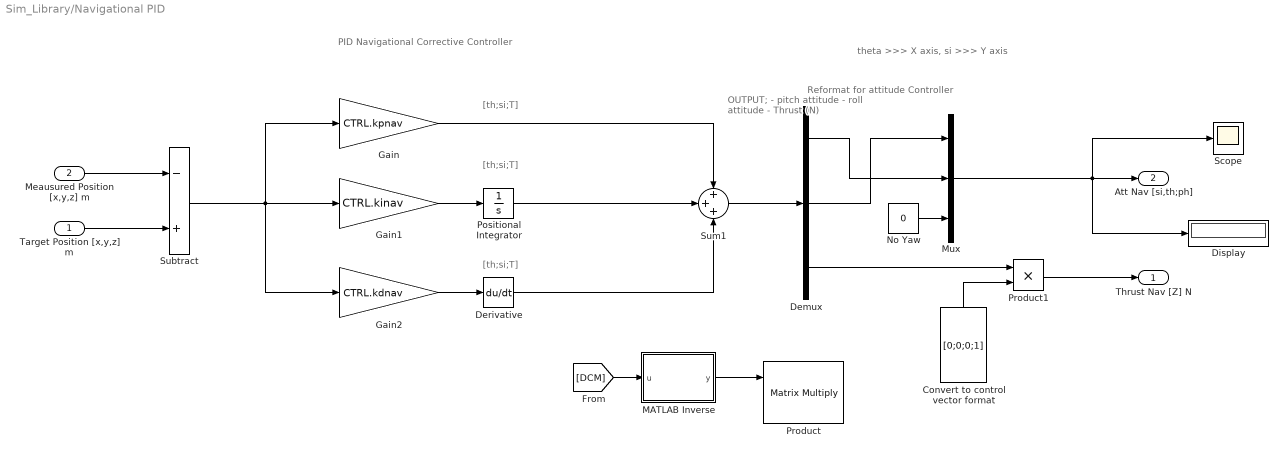
== system Sim_Library/Navigational PID ==
  note: Reformat for attitude Controller
  note: theta >>> X axis, si >>> Y axis
  note: [th;si;T]
  note: OUTPUT;
      | - pitch attitude
      | - roll attitude
      | - Thrust (N)
  note: PID Navigational Corrective Controller
  note: [th;si;T]
  note: [th;si;T]
  Target Position [x,y,z] m : Inport
  Meausured Position [x,y,z] m : Inport  Port=2
  Convert to control vector format : Constant  Value=[0;0;0;1]  VectorParams1D=off
  Demux : Demux  Outputs=3
  Derivative : Derivative
  Display : Display
  Gain : Gain  Gain=CTRL.kpnav
  Gain1 : Gain  Gain=CTRL.kinav
  Gain2 : Gain  Gain=CTRL.kdnav
  MATLAB Inverse : MATLAB Function  TreatAsAtomicUnit=on
  Mux : Mux  Inputs=3
  No Yaw : Constant  Value=0
  Positional Integrator : Integrator
  Product : Product  Multiplication=Matrix(*)
  Product1 : Product
  Scope : Scope
  Subtract : Sum  Inputs=-+
  Sum1 : Sum  Inputs=+++
  Thrust Nav [Z] N : Outport
  Att Nav [si,th;ph] : Outport  Port=2
  wires:
  Derivative/1 -> Sum1/3
  Gain2/1 -> Derivative/1
  Subtract/1 -> Gain1/1, Gain/1, Gain2/1
  Positional Integrator/1 -> Sum1/2
  Gain1/1 -> Positional Integrator/1
  Target Position [x,y,z] m/1 -> Subtract/2
  Meausured Position [x,y,z] m/1 -> Subtract/1
  Gain/1 -> Sum1/1
  Sum1/1 -> Demux/1
  Mux/1 -> Display/1, Att Nav [si,th;ph]/1, Scope/1
  [DCM] -> MATLAB Inverse/1(u)
  MATLAB Inverse/1(y) -> Product/1
  Demux/2 -> Mux/1
  Demux/1 -> Mux/2
  No Yaw/1 -> Mux/3
  Demux/3 -> Product1/1
  Convert to control vector format/1 -> Product1/2
  Product1/1 -> Thrust Nav [Z] N/1

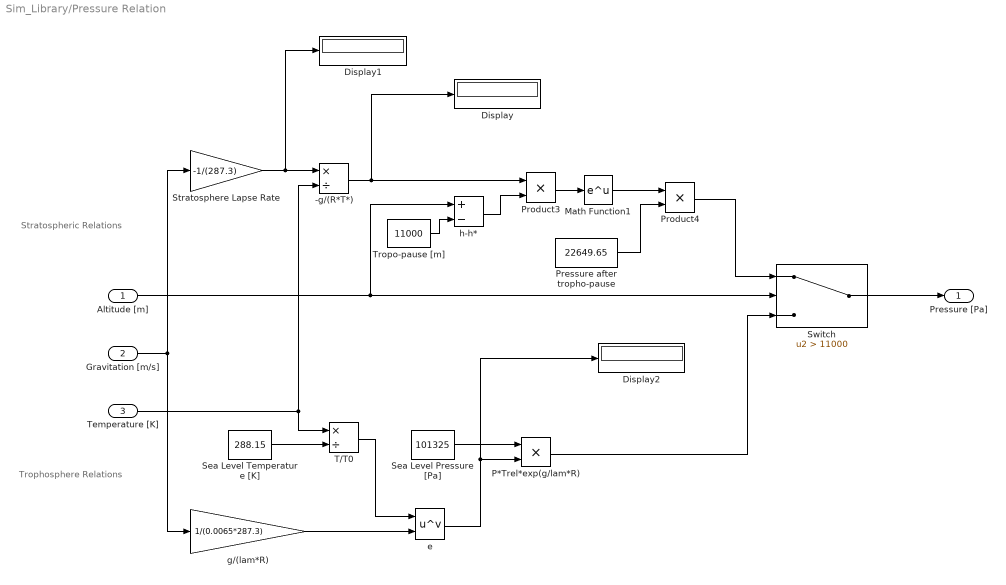
== system Sim_Library/Pressure Relation ==
  note: Stratospheric Relations
  note: Trophosphere Relations
  Altitude [m] : Inport
  Gravitation [m/s] : Inport  Port=2
  Temperature [K] : Inport  Port=3
  -g/(R*T*) : Product  Inputs=*/
  Display : Display
  Display1 : Display
  Display2 : Display
  Math Function1 : Math  SaturateOnIntegerOverflow=on
  P*Trel*exp(g/lam*R) : Product
  Pressure after tropho-pause : Constant  Value=22649.65
  Product3 : Product
  Product4 : Product
  Sea Level Temperature [K] : Constant  Value=288.15
  Sea Level Pressure [Pa] : Constant  Value=101325
  Stratosphere Lapse Rate : Gain  Gain=-1/(287.3)
  Switch : Switch  Criteria=u2 > Threshold  Threshold=11000
  T/T0 : Product  Inputs=*/
  Tropo-pause [m] : Constant  Value=11000
  e : Math  Operator=pow  SaturateOnIntegerOverflow=on
  g/(lam*R) : Gain  Gain=1/(0.0065*287.3)
  h-h* : Sum  Inputs=+-
  Pressure [Pa] : Outport
  wires:
  g/(lam*R)/1 -> e/2
  T/T0/1 -> e/1
  Product4/1 -> Switch/1
  Pressure after tropho-pause/1 -> Product4/2
  Math Function1/1 -> Product4/1
  Product3/1 -> Math Function1/1
  h-h*/1 -> Product3/2
  -g/(R*T*)/1 -> Product3/1, Display/1
  Tropo-pause [m]/1 -> h-h*/2
  Stratosphere Lapse Rate/1 -> -g/(R*T*)/1, Display1/1
  P*Trel*exp(g/lam*R)/1 -> Switch/3
  e/1 -> P*Trel*exp(g/lam*R)/2, Display2/1
  Sea Level Pressure [Pa]/1 -> P*Trel*exp(g/lam*R)/1
  Sea Level Temperature [K]/1 -> T/T0/2
  Temperature [K]/1 -> -g/(R*T*)/2, T/T0/1
  Gravitation [m/s]/1 -> Stratosphere Lapse Rate/1, g/(lam*R)/1
  Altitude [m]/1 -> Switch/2, h-h*/1
  Switch/1 -> Pressure [Pa]/1

== system Sim_Library/Quadrotor (+ - x) Gyro Mapping ==
  note: Rotors 1 & 3 Negative
  Rotor Velocities [w1;w2;w3;w4] : Inport
  Constant : Constant  Value=[0;0;1]  VectorParams1D=off
  Demux : Demux
  Product : Product  Multiplication=Matrix(*)
  Product1 : Product
  Rotor Inertia : Constant  Value=agent.rotor.I
  Sum : Sum  Inputs=+-+-
  " Gyroscopic Momentum [Jx;Jy;Jz]" : Outport
  wires:
  Product/1 -> " Gyroscopic Momentum [Jx;Jy;Jz]"/1
  Product1/1 -> Product/2
  Rotor Inertia/1 -> Product/1
  Sum/1 -> Product1/1
  Demux/4 -> Sum/4
  Demux/3 -> Sum/3
  Demux/2 -> Sum/2
  Demux/1 -> Sum/1
  Constant/1 -> Product1/2
  Rotor Velocities [w1;w2;w3;w4]/1 -> Demux/1

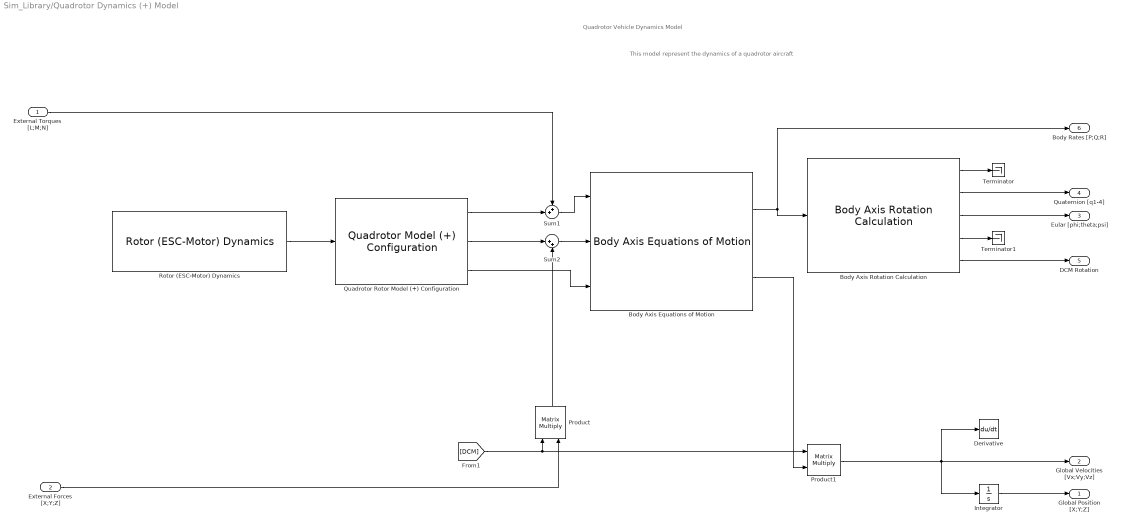
== system Sim_Library/Quadrotor Dynamics (+) Model ==
  note: This model represent the dynamics of a quadrotor aircraft
  note: Quadrotor Vehicle Dynamics Model
  External Torques [L;M;N] : Inport
  External Forces [X;Y;Z] : Inport  Port=2
  Body Axis Equations of Motion : Sim_Library/Body Axis Equations of Motion  SystemSampleTime=-1
  "Body Axis Rotation Calculation " : Sim_Library/Body Axis Rotation Calculation   SystemSampleTime=-1
  Derivative : Derivative
  Integrator : Integrator  InitialCondition=[0;0;0]
  Product : Product  Multiplication=Matrix(*)
  Product1 : Product  Multiplication=Matrix(*)
  Quadrotor Rotor Model (+) Configuration : Sim_Library/Quadrotor Model (+) Configuration  SystemSampleTime=-1
  Rotor (ESC-Motor) Dynamics : Sim_Library/Rotor (ESC-Motor) Dynamics  SystemSampleTime=-1
  Sum1 : Sum  Inputs=++|
  Sum2 : Sum  Inputs=|++
  Terminator : Terminator
  Terminator1 : Terminator
  Global Position [X;Y;Z] : Outport
  Global Velocities [Vx;Vy;Vz] : Outport  Port=2
  Eular [phi;theta;psi] : Outport  Port=3
  Quaternion [q1-4] : Outport  Port=4
  DCM Rotation : Outport  Port=5
  Body Rates [P;Q;R] : Outport  Port=6
  wires:
  [DCM] -> Product/1, Product1/1
  External Forces [X;Y;Z]/1 -> Product/2
  Rotor (ESC-Motor) Dynamics/1 -> Quadrotor Rotor Model (+) Configuration/1
  Quadrotor Rotor Model (+) Configuration/1 -> Sum1/2
  Sum1/1 -> Body Axis Equations of Motion/1
  Sum2/1 -> Body Axis Equations of Motion/2
  External Torques [L;M;N]/1 -> Sum1/1
  Quadrotor Rotor Model (+) Configuration/2 -> Sum2/1
  Product/1 -> Sum2/2
  Body Axis Equations of Motion/1 -> "Body Axis Rotation Calculation "/1, Body Rates [P;Q;R]/1
  "Body Axis Rotation Calculation "/3 -> Eular [phi;theta;psi]/1
  "Body Axis Rotation Calculation "/5 -> DCM Rotation/1
  Body Axis Equations of Motion/2 -> Product1/2
  Product1/1 -> Derivative/1, Integrator/1, Global Velocities [Vx;Vy;Vz]/1
  "Body Axis Rotation Calculation "/2 -> Quaternion [q1-4]/1
  "Body Axis Rotation Calculation "/1 -> Terminator/1
  "Body Axis Rotation Calculation "/4 -> Terminator1/1
  Integrator/1 -> Global Position [X;Y;Z]/1
  Quadrotor Rotor Model (+) Configuration/3 -> Body Axis Equations of Motion/3

== system Sim_Library/Quadrotor Manual Control  ==
  note: U3
  note: U1
  note: This Subsystem is designed to map the controllers inputs and command inputs onto the rotors outputs
  note: Control Output Signal Map- (+) Configuration
  note: U2
  note: U4
  User Inputs [U1;U2;U3;U4] : Inport
  Demux : Demux
  Display : Display
  Mux : Mux
  Saturation : Saturate  UpperLimit=255  LowerLimit=0
  Saturation Limits : Saturate  UpperLimit=255  LowerLimit=0
  Saturation1 : Saturate  UpperLimit=255  LowerLimit=0
  Saturation2 : Saturate  UpperLimit=255  LowerLimit=0
  Sum1 : Sum  Inputs=+++
  Sum2 : Sum  Inputs=+--
  Sum3 : Sum  Inputs=+-+
  Sum4 : Sum  Inputs=++-
  Servo Set points [S1;S2;S3;S4] : Outport
  wires:
  Mux/1 -> Servo Set points [S1;S2;S3;S4]/1, Display/1
  User Inputs [U1;U2;U3;U4]/1 -> Demux/1
  Saturation/1 -> Mux/1
  Saturation1/1 -> Mux/2
  Saturation2/1 -> Mux/3
  Saturation Limits/1 -> Mux/4
  Sum1/1 -> Saturation/1
  Sum2/1 -> Saturation1/1
  Sum3/1 -> Saturation2/1
  Sum4/1 -> Saturation Limits/1
  Demux/1 -> Sum1/1, Sum2/1, Sum3/1, Sum4/1
  Demux/2 -> Sum4/2, Sum2/2
  Demux/3 -> Sum1/2, Sum3/2
  Demux/4 -> Sum3/3, Sum2/3, Sum1/3, Sum4/3

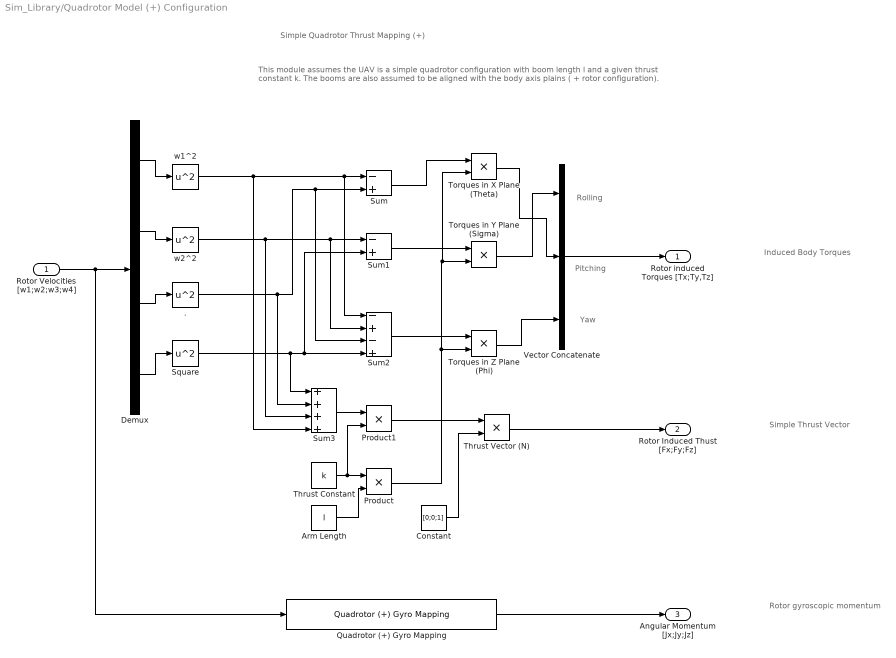
== system Sim_Library/Quadrotor Model (+) Configuration ==
  note: Induced Body Torques
  note: Simple Thrust Vector
  note: Simple Quadrotor Thrust Mapping (+)
  note: Pitching
  note: Rolling
  note: Yaw
  note: This module assumes the UAV is a simple quadrotor configuration with boom length l and a given thrust constant k.
      | The booms are also assumed to be aligned with the body axis plains ( + rotor configuration).
  note: Rotor gyroscopic momentum
  Rotor Velocities [w1;w2;w3;w4] : Inport
  . : Math  Operator=square  SaturateOnIntegerOverflow=on
  Arm Length : Constant  Value=l
  Constant : Constant  Value=[0;0;1]  VectorParams1D=off
  Demux : Demux
  Product : Product
  Product1 : Product
  Quadrotor (+) Gyro Mapping : Sim_Library/Quadrotor (+) Gyro Mapping  SystemSampleTime=-1
  "Square " : Math  Operator=square  SaturateOnIntegerOverflow=on
  Sum : Sum  Inputs=-+
  Sum1 : Sum  Inputs=-+
  Sum2 : Sum  Inputs=-+-+
  Sum3 : Sum  Inputs=++++
  Thrust Constant : Constant  Value=k
  Thrust Vector (N) : Product
  Torques in X Plane (Theta) : Product
  Torques in Y Plane (Sigma) : Product
  Torques in Z Plane (Phi) : Product
  Vector Concatenate : Concatenate  NumInputs=3  Mode=Multidimensional array
  w1^2 : Math  Operator=square  SaturateOnIntegerOverflow=on
  w2^2 : Math  Operator=square  SaturateOnIntegerOverflow=on
  Rotor induced Torques [Tx;Ty,Tz] : Outport
  Rotor Induced Thust [Fx;Fy;Fz] : Outport  Port=2
  Angular Momentum [Jx;Jy;Jz] : Outport  Port=3
  wires:
  Thrust Vector (N)/1 -> Rotor Induced Thust [Fx;Fy;Fz]/1
  Vector Concatenate/1 -> Rotor induced Torques [Tx;Ty,Tz]/1
  Demux/3 -> ./1
  Demux/1 -> w1^2/1
  Demux/4 -> "Square "/1
  Rotor Velocities [w1;w2;w3;w4]/1 -> Quadrotor (+) Gyro Mapping/1, Demux/1
  Torques in X Plane (Theta)/1 -> Vector Concatenate/2
  Torques in Z Plane (Phi)/1 -> Vector Concatenate/3
  Torques in Y Plane (Sigma)/1 -> Vector Concatenate/1
  Constant/1 -> Thrust Vector (N)/2
  Product1/1 -> Thrust Vector (N)/1
  ./1 -> Sum/2, Sum2/3, Sum3/2
  Sum/1 -> Torques in X Plane (Theta)/1
  Sum1/1 -> Torques in Y Plane (Sigma)/1
  Product/1 -> Torques in Z Plane (Phi)/2, Torques in Y Plane (Sigma)/2, Torques in X Plane (Theta)/2
  Arm Length/1 -> Product/2
  Sum3/1 -> Product1/1
  w1^2/1 -> Sum/1, Sum2/1, Sum3/4
  Thrust Constant/1 -> Product/1, Product1/2
  w2^2/1 -> Sum1/1, Sum2/2, Sum3/3
  Sum2/1 -> Torques in Z Plane (Phi)/1
  "Square "/1 -> Sum1/2, Sum2/4, Sum3/1
  Demux/2 -> w2^2/1
  Quadrotor (+) Gyro Mapping/1 -> Angular Momentum [Jx;Jy;Jz]/1

== system Sim_Library/Quaternion to 3x3 DCM  ==
  note: Quaternions >> DCM Rotation Matrix
  "Quaternion [q0,q1,q2,q3] " : Inport
  Create 3x3 Matrix : aerolibutil/Create 3x3 Matrix
  element AA : Fcn  Expr=(u(1)^2)-(u(2)^2)-(u(3)^2)+(u(4)^2)
  element AB : Fcn  Expr=2*(u(1)*u(2)+u(1)*u(4))
  element AC : Fcn  Expr=2*(u(1)*u(3)-u(2)*u(4))
  element BA : Fcn  Expr=2*(u(1)*u(2)-u(3)*u(4))
  element BB : Fcn  Expr=-u(1)^2+u(2)^2-u(3)^2+u(4)^2
  element BC : Fcn  Expr=2*(u(2)*u(3)+u(1)*u(4))
  element CA : Fcn  Expr=2*(u(1)*u(3)+u(2)*u(4))
  element CB : Fcn  Expr=2*(u(2)*u(3)-u(1)*u(4))
  element CC : Fcn  Expr=-(u(1)^2)-(u(2)^2)+(u(3)^2)+(u(4)^2)
  3x3 DCM Rotation : Outport
  wires:
  "Quaternion [q0,q1,q2,q3] "/1 -> element BC/1, element CC/1, element CB/1, element CA/1, element AC/1, element AB/1, element AA/1, element BA/1, element BB/1
  element CB/1 -> Create 3x3 Matrix/8
  element AA/1 -> Create 3x3 Matrix/1
  element AB/1 -> Create 3x3 Matrix/2
  element BA/1 -> Create 3x3 Matrix/4
  element AC/1 -> Create 3x3 Matrix/3
  element BC/1 -> Create 3x3 Matrix/6
  element CC/1 -> Create 3x3 Matrix/9
  element BB/1 -> Create 3x3 Matrix/5
  element CA/1 -> Create 3x3 Matrix/7
  Create 3x3 Matrix/1 -> 3x3 DCM Rotation/1

== system Sim_Library/Quaternion to Eular Angles ==
  note: Quaternions >> Eular Angles
  note: sigma
  note: phi
  note: phi
  "Quaternion [q0,q1,q2,q3] " : Inport
  Display : Display
  Gain : Gain  Gain=180/pi
  Phi Denominator : Fcn  Expr=u(1)^2-u(2)^2-u(3)^2+u(4)^2
  Phi Numerator : Fcn  Expr=2*(u(1)*u(2)+u(3)*u(4))
  Si Denominator : Fcn  Expr=-u(1)^2-u(2)^2+u(3)^2+u(4)^2
  Si numerator : Fcn  Expr=2*(u(2)*u(3)+u(1)*u(4))
  Theta Numerator (no dom) : Fcn  Expr=-2*(u(1)*u(3)-u(2)*u(4))
  Trigonometric Function : Trigonometry  Operator=asin
  Trigonometric Function1 : Trigonometry  Operator=atan2
  Trigonometric Function2 : Trigonometry  Operator=atan2
  Vector Concatenate : Concatenate  NumInputs=3  Mode=Multidimensional array
  Eular Angle [si,the,phi] : Outport
  wires:
  "Quaternion [q0,q1,q2,q3] "/1 -> Theta Numerator (no dom)/1, Si numerator/1, Si Denominator/1, Phi Numerator/1, Phi Denominator/1
  Si numerator/1 -> Trigonometric Function1/1
  Si Denominator/1 -> Trigonometric Function1/2
  Gain/1 -> Display/1
  Trigonometric Function2/1 -> Vector Concatenate/3
  Phi Denominator/1 -> Trigonometric Function2/2
  Phi Numerator/1 -> Trigonometric Function2/1
  Trigonometric Function1/1 -> Vector Concatenate/1
  Vector Concatenate/1 -> Eular Angle [si,the,phi]/1, Gain/1
  Theta Numerator (no dom)/1 -> Trigonometric Function/1
  Trigonometric Function/1 -> Vector Concatenate/2

== system Sim_Library/Rear Stabiliser ==
  In1 : Inport
  Out1 : Outport
  wires:
  In1/1 -> Out1/1

== system Sim_Library/Relative Gravitational Magnitude ==
  note: Acceleration as a
      | global constant
  note: Assumptions; Gravitational linearity, reference is Earth and down is positive.
  note: Newtons equation of gravity, extended to provide a local gravitational vector
  note: Gravitational Model
  Altitude [m] : Inport
  Divide : Product  Inputs=*/
  Gravitational Constant [Nm^2/kg^2] : Constant  Value=6.673*10^-11  VectorParams1D=off
  Mass Of The Earth [kg] : Constant  Value=5.972*10^24  VectorParams1D=off
  Math Function : Math  Operator=square  SaturateOnIntegerOverflow=on
  Product : Product
  Radius of The Earth [m] : Constant  Value=6371*10^3  VectorParams1D=off
  Sum : Sum  Inputs=|++
  Local Accel [m/s] : Outport
  wires:
  Gravitational Constant [Nm^2/kg^2]/1 -> Product/1
  Mass Of The Earth [kg]/1 -> Product/2
  Altitude [m]/1 -> Sum/1
  Radius of The Earth [m]/1 -> Sum/2
  Sum/1 -> Math Function/1
  Product/1 -> Divide/1
  Math Function/1 -> Divide/2
  Divide/1 -> Local Accel [m/s]/1

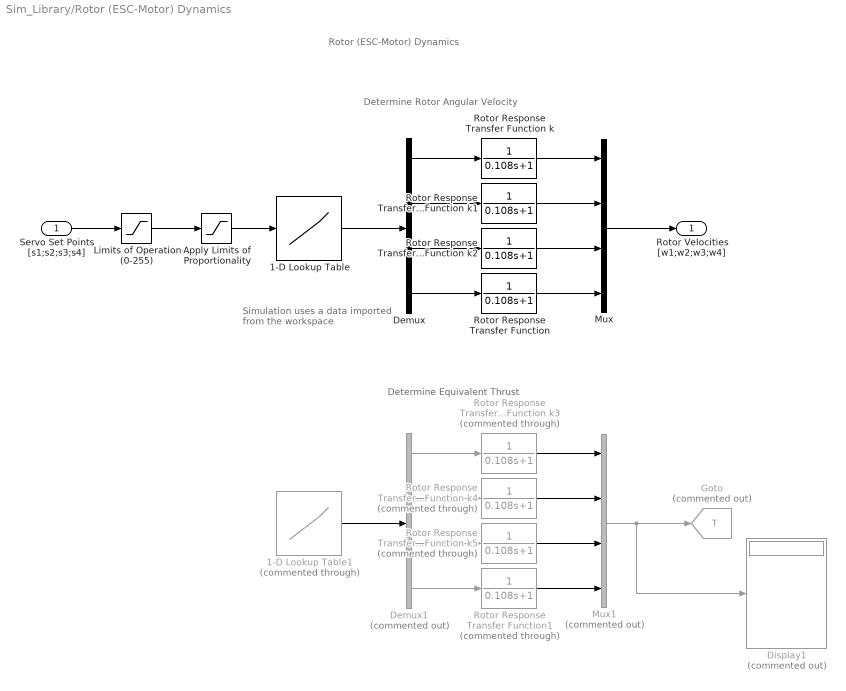
== system Sim_Library/Rotor (ESC-Motor) Dynamics ==
  note: Simulation uses a data
      | imported from the workspace
  note: Determine Equivalent Thrust
  note: Determine Rotor Angular Velocity
  note: Rotor (ESC-Motor) Dynamics
  Servo Set Points [s1;s2;s3;s4] : Inport
  1-D Lookup Table : Lookup_n-D  NumberOfTableDimensions=1  BreakpointsForDimension1=[0:255]  Table=ROTOR.angVdata  ExtrapMethod=Clip  UseLastTableValue=on  InternalRulePriority=Speed  RndMeth=Simplest  InputSameDT=on
  1-D Lookup Table1 : Lookup_n-D  Commented=through  NumberOfTableDimensions=1  BreakpointsForDimension1=[0:255]  Table=ROTOR.ThrNdata  ExtrapMethod=Clip  UseLastTableValue=on  InternalRulePriority=Speed  RndMeth=Simplest  InputSameDT=on
  Apply Limits of Proportionality : Saturate  UpperLimit=117  LowerLimit=27  ZeroCross=off
  Demux : Demux
  Demux1 : Demux  Commented=on
  Display1 : Display  Commented=on
  Goto : Goto  Commented=on  GotoTag=T  TagVisibility=global
  Limits of Operation (0-255) : Saturate  UpperLimit=255  LowerLimit=0  ZeroCross=off
  Mux : Mux
  Mux1 : Mux  Commented=on
  Rotor Response Transfer Function : TransferFcn  Denominator=[0.108 1]
  Rotor Response Transfer Function k : TransferFcn  Denominator=[0.108 1]
  Rotor Response Transfer Function k1 : TransferFcn  Denominator=[0.108 1]
  Rotor Response Transfer Function k2 : TransferFcn  Denominator=[0.108 1]
  Rotor Response Transfer Function k3 : TransferFcn  Commented=through  Denominator=[0.108 1]
  Rotor Response Transfer Function k4 : TransferFcn  Commented=through  Denominator=[0.108 1]
  Rotor Response Transfer Function k5 : TransferFcn  Commented=through  Denominator=[0.108 1]
  Rotor Response Transfer Function1 : TransferFcn  Commented=through  Denominator=[0.108 1]
  Rotor Velocities [w1;w2;w3;w4] : Outport
  wires:
  1-D Lookup Table1/1 -> Demux1/1
  Mux1/1 -> Display1/1, Goto/1
  1-D Lookup Table/1 -> Demux/1
  Rotor Response Transfer Function1/1 -> Mux1/4
  Rotor Response Transfer Function k5/1 -> Mux1/3
  Rotor Response Transfer Function k4/1 -> Mux1/2
  Rotor Response Transfer Function k3/1 -> Mux1/1
  Demux1/4 -> Rotor Response Transfer Function1/1
  Demux1/3 -> Rotor Response Transfer Function k5/1
  Demux1/2 -> Rotor Response Transfer Function k4/1
  Demux1/1 -> Rotor Response Transfer Function k3/1
  Mux/1 -> Rotor Velocities [w1;w2;w3;w4]/1
  Rotor Response Transfer Function/1 -> Mux/4
  Rotor Response Transfer Function k2/1 -> Mux/3
  Rotor Response Transfer Function k1/1 -> Mux/2
  Rotor Response Transfer Function k/1 -> Mux/1
  Demux/4 -> Rotor Response Transfer Function/1
  Demux/3 -> Rotor Response Transfer Function k2/1
  Demux/2 -> Rotor Response Transfer Function k1/1
  Demux/1 -> Rotor Response Transfer Function k/1
  Apply Limits of Proportionality/1 -> 1-D Lookup Table/1
  Limits of Operation (0-255)/1 -> Apply Limits of Proportionality/1
  Servo Set Points [s1;s2;s3;s4]/1 -> Limits of Operation (0-255)/1

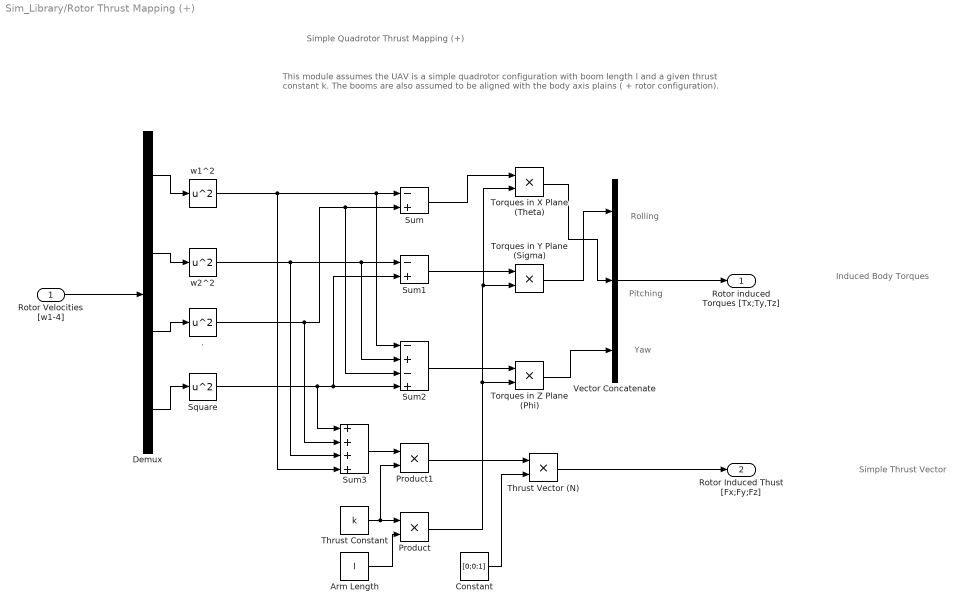
== system Sim_Library/Rotor Thrust Mapping (+) ==
  note: Induced Body Torques
  note: Simple Thrust Vector
  note: Simple Quadrotor Thrust Mapping (+)
  note: Pitching
  note: Rolling
  note: Yaw
  note: This module assumes the UAV is a simple quadrotor configuration with boom length l and a given thrust constant k.
      | The booms are also assumed to be aligned with the body axis plains ( + rotor configuration).
  Rotor Velocities [w1-4] : Inport
  . : Math  Operator=square  SaturateOnIntegerOverflow=on
  Arm Length : Constant  Value=l
  Constant : Constant  Value=[0;0;1]  VectorParams1D=off
  Demux : Demux
  Product : Product
  Product1 : Product
  "Square " : Math  Operator=square  SaturateOnIntegerOverflow=on
  Sum : Sum  Inputs=-+
  Sum1 : Sum  Inputs=-+
  Sum2 : Sum  Inputs=-+-+
  Sum3 : Sum  Inputs=++++
  Thrust Constant : Constant  Value=k
  Thrust Vector (N) : Product
  Torques in X Plane (Theta) : Product
  Torques in Y Plane (Sigma) : Product
  Torques in Z Plane (Phi) : Product
  Vector Concatenate : Concatenate  NumInputs=3  Mode=Multidimensional array
  w1^2 : Math  Operator=square  SaturateOnIntegerOverflow=on
  w2^2 : Math  Operator=square  SaturateOnIntegerOverflow=on
  Rotor induced Torques [Tx;Ty,Tz] : Outport
  Rotor Induced Thust [Fx;Fy;Fz] : Outport  Port=2
  wires:
  Thrust Vector (N)/1 -> Rotor Induced Thust [Fx;Fy;Fz]/1
  Vector Concatenate/1 -> Rotor induced Torques [Tx;Ty,Tz]/1
  Demux/3 -> ./1
  Demux/1 -> w1^2/1
  Demux/4 -> "Square "/1
  Rotor Velocities [w1-4]/1 -> Demux/1
  Torques in X Plane (Theta)/1 -> Vector Concatenate/2
  Torques in Z Plane (Phi)/1 -> Vector Concatenate/3
  Torques in Y Plane (Sigma)/1 -> Vector Concatenate/1
  Constant/1 -> Thrust Vector (N)/2
  Product1/1 -> Thrust Vector (N)/1
  ./1 -> Sum/2, Sum2/3, Sum3/2
  Sum/1 -> Torques in X Plane (Theta)/1
  Sum1/1 -> Torques in Y Plane (Sigma)/1
  Product/1 -> Torques in Z Plane (Phi)/2, Torques in Y Plane (Sigma)/2, Torques in X Plane (Theta)/2
  Arm Length/1 -> Product/2
  Sum3/1 -> Product1/1
  w1^2/1 -> Sum/1, Sum2/1, Sum3/4
  Thrust Constant/1 -> Product/1, Product1/2
  w2^2/1 -> Sum1/1, Sum2/2, Sum3/3
  Sum2/1 -> Torques in Z Plane (Phi)/1
  "Square "/1 -> Sum1/2, Sum2/4, Sum3/1
  Demux/2 -> w2^2/1
